simulink model "SimulinkModel"  (R2025b)
settings: Solver=VariableStepAuto  StartTime=0.0  StopTime=3600  FixedStep=0.1  MaxStep=5  MinStep=1  RelTol=0.5e-5  AbsTol=1e-5
values from neighbouring files (symbols this model uses):
  clock_drift_rate = 0.5    [run_simulink.m]    (also in sat_scenario.m)
undefined symbols (not defined in the file or in its folder): accelCorrectionInterval, baroCorrectionInterval, deg, gpsCorrectionInterval, IAU, IMUPropInterval, magCorrectionInterval, R_vec, rad, s, WMM2025
libraries: aerolibtransform2 x6, aerolibconvert2 x2, aerolibutil x2, aerolibsatdyn x1, aerolibnav x1, aerolibgravity2 x1, vrlib x1
settings Model: Creator=abhay  LastModifiedBy=abhay
settings DataIOCC: DatasetSignalFormat=timetable

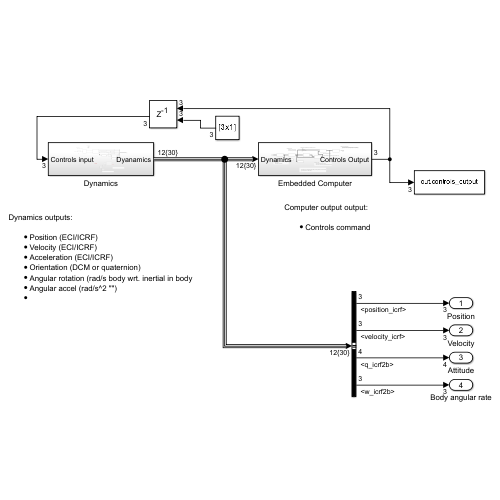
[thumbnail: Simulink's stored preview of the top-level diagram]
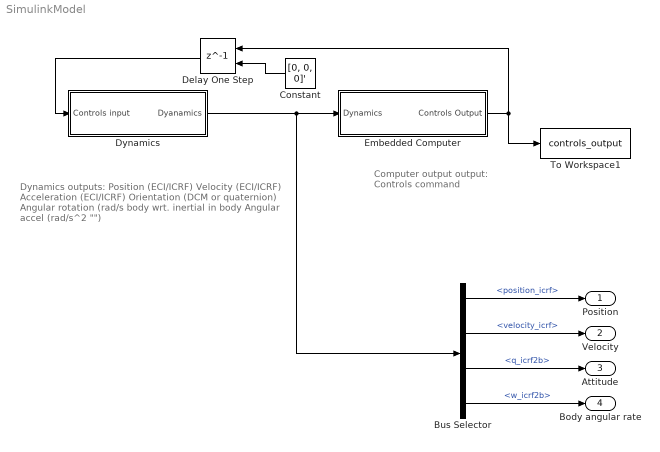
== system SimulinkModel ==
  note: Dynamics outputs:
      |
      | Position (ECI/ICRF)
      | Velocity (ECI/ICRF)
      | Acceleration (ECI/ICRF)
      | Orientation (DCM or quaternion)
      | Angular rotation (rad/s body wrt. inertial in body
      | Angular accel (rad/s^2 "")
  note: Computer output output:
      |
      | Controls command
  Bus Selector : BusSelector  OutputSignals=position_icrf,velocity_icrf,q_icrf2b,w_icrf2b
  Constant : Constant  Value=[0, 0, 0]'
  Delay One Step : Delay  DelayLength=1  InitialConditionSource=Input port
      settings: InputPortMap=u0,p4
  Dynamics : Subsystem
  Embedded Computer : Subsystem
  To Workspace1 : ToWorkspace  VariableName=controls_output  SaveFormat=Timeseries  SampleTime=-1
  Position : Outport
  Velocity : Outport  Port=2
  Attitude : Outport  Port=3
  Body angular rate : Outport  Port=4
  wires:
  Dynamics/1(Dyanamics) -> Bus Selector/1, Embedded Computer/1(Dynamics)
  Embedded Computer/1(Controls Output) -> Delay One Step/1, To Workspace1/1
  Delay One Step/1 -> Dynamics/1(Controls input)
  Constant/1 -> Delay One Step/2
  Bus Selector/1 -> Position/1  "<position_icrf>"
  Bus Selector/2 -> Velocity/1  "<velocity_icrf>"
  Bus Selector/3 -> Attitude/1  "<q_icrf2b>"
  Bus Selector/4 -> Body angular rate/1  "<w_icrf2b>"

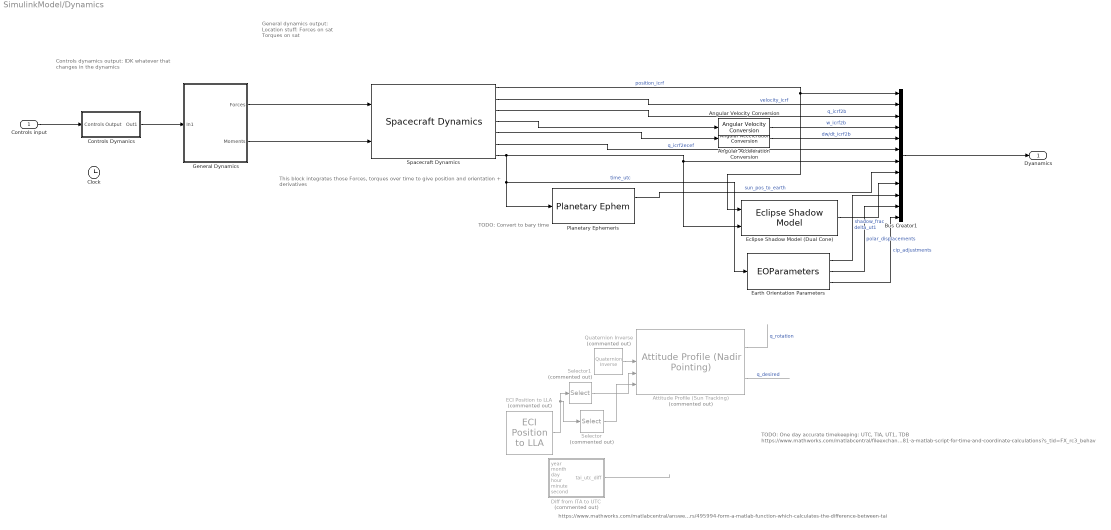
== system SimulinkModel/Dynamics ==
  note: TODO: One day accurate timekeeping: UTC, TIA, UT1, TDB
      |
      | https://www.mathworks.com/matlabcentral/fileexchange/41681-a-matlab-script-for-time-and-coordinate-calculations?s_tid=FX_rc3_behav
  note: TODO: Convert to bary time
  note: https://www.mathworks.com/matlabcentral/answers/495994-form-a-matlab-function-which-calculates-the-difference-between-tai
  note: This block integrates those Forces, torques over time to give position and orientation
      | + derivatives
  note: Controls dynamics output:
      |
      | IDK whatever that changes in the dynamics
  note: General dynamics output:
      |
      | Location stuff:
      | Forces on sat
      | Torques on sat
  Controls input : Inport
  Angular Acceleration Conversion : aerolibconvert2/Angular Acceleration Conversion  IU=deg/s^2  OU=rad/s^2
  Angular Velocity Conversion : aerolibconvert2/Angular Velocity Conversion  IU=deg/s  OU=rad/s
  Attitude Profile (Sun Tracking) : aerolibsatdyn/Attitude Profile (Nadir Pointing)  Commented=on  outputError=on  outputFinalAttitude=on  portFrame=ICRF  pointingMode=Point at celestial body  celestialTarget=Sun  tunablePointing=on  primaryAlignmentSrc=Dialog  primaryAlignment=[0 0 1]  secondaryAlignmentSrc=Dialog  secondaryAlignment=[1 0 0]  constraintFrame=ICRF  primaryConstraintSrc=Dialog  primaryConstraint=[1 0 0]  secondaryConstraintSrc=Dialog  secondaryConstraint=[0 1 0]
      settings: LibrarySourceBlock=|
      | aerolibsatdyn/Attitude Profile
      | (Sun Tracking)
  Bus Creator1 : BusCreator  Inputs=12
  Clock : Clock
  Controls Dymanics : Subsystem
  "Diff from ITA to UTC  " : MATLAB Function  Commented=on  TreatAsAtomicUnit=on
  ECI Position to LLA : aerolibtransform2/ECI Position to LLA  Commented=on  red=IAU-2000/2006  year=2013  month=January  day=1  hour=0  min=0  sec=0  deltaT=Day  errorflag=Error  extraparamflag=on  eunits=Metric (MKS)  earthmodel=WGS84  flat=1/298.257223563  eqradius=6378137
      settings: AttributesFormatString=%<red>
  Earth Orientation Parameters : EOParameters
  Eclipse Shadow Model (Dual Cone) : EclipseShadowModel  timeSource=Port (Julian date)  useEphemerisDateRange=off  zeroCrossing=on
  General Dynamics : Subsystem
  Planetary Ephemeris : PlanetaryEphem  units=m,m/s  target=Sun
  Quaternion Inverse : aerolibutil/Quaternion Inverse  Commented=on
  Selector : Selector  Commented=on  InputPortWidth=3  IndexOptions=Index vector (dialog)  Indices=[3]  OutputSizes=1
  Selector1 : Selector  Commented=on  InputPortWidth=3  IndexOptions=Index vector (dialog)  Indices=[1 2]  OutputSizes=1
  Spacecraft Dynamics : SpacecraftDynamics  startDate=2459581  mass=0.250  inertia=inertia_tensor  semiMajorAxis=6865000  eccentricity=0.0002105  inclination=97.4  raan=0  argPeriapsis=0  trueAnomaly=0  attitude=[0.263360579192421 0.571813128030932 0.494678363680335 0.599136268678053]  attitudeRate=[10 5 2.5]  outputAngAccel=on  outputTransform=on  useDrag=on  useEphemerisDateRange=off  useSRP=on
  Dyanamics : Outport
  wires:
  Controls Dymanics/1(Out1) -> General Dynamics/1(In1)
  General Dynamics/1(Forces) -> Spacecraft Dynamics/1
  General Dynamics/2(Moments) -> Spacecraft Dynamics/2
  Spacecraft Dynamics/1 -> Eclipse Shadow Model (Dual Cone)/1, Bus Creator1/1  "position_icrf"
  Spacecraft Dynamics/2 -> Bus Creator1/2  "velocity_icrf"
  Spacecraft Dynamics/3 -> Bus Creator1/3  "q_icrf2b"
  Spacecraft Dynamics/4 -> Angular Velocity Conversion/1
  Spacecraft Dynamics/5 -> Angular Acceleration Conversion/1
  Spacecraft Dynamics/6 -> Bus Creator1/6  "q_icrf2ecef"
  Spacecraft Dynamics/7 -> Eclipse Shadow Model (Dual Cone)/2, Bus Creator1/7, Planetary Ephemeris/1, Earth Orientation Parameters/1  "time_utc"
  Bus Creator1/1 -> Dyanamics/1
  Controls input/1 -> Controls Dymanics/1(Controls Output)
  ? -> ?
  Angular Velocity Conversion/1 -> Bus Creator1/4  "w_icrf2b"
  Angular Acceleration Conversion/1 -> Bus Creator1/5  "dw/dt_icrf2b"
  Quaternion Inverse/1 -> Attitude Profile (Sun Tracking)/3
  Planetary Ephemeris/1 -> Bus Creator1/8  "sun_pos_to_earth"
  Selector/1 -> Attitude Profile (Sun Tracking)/5
  ECI Position to LLA/1 -> Selector1/1, Selector/1
  Selector1/1 -> Attitude Profile (Sun Tracking)/4
  Attitude Profile (Sun Tracking)/1 -> ?  "q_rotation"
  Attitude Profile (Sun Tracking)/2 -> ?  "q_desired"
  "Diff from ITA to UTC  "/1(tai_utc_diff) -> ?
  Eclipse Shadow Model (Dual Cone)/1 -> Bus Creator1/9  "shadow_frac"
  Earth Orientation Parameters/1 -> Bus Creator1/10  "delta_ut1"
  Earth Orientation Parameters/2 -> Bus Creator1/11  "polar_displacements"
  Earth Orientation Parameters/3 -> Bus Creator1/12  "cip_adjustments"

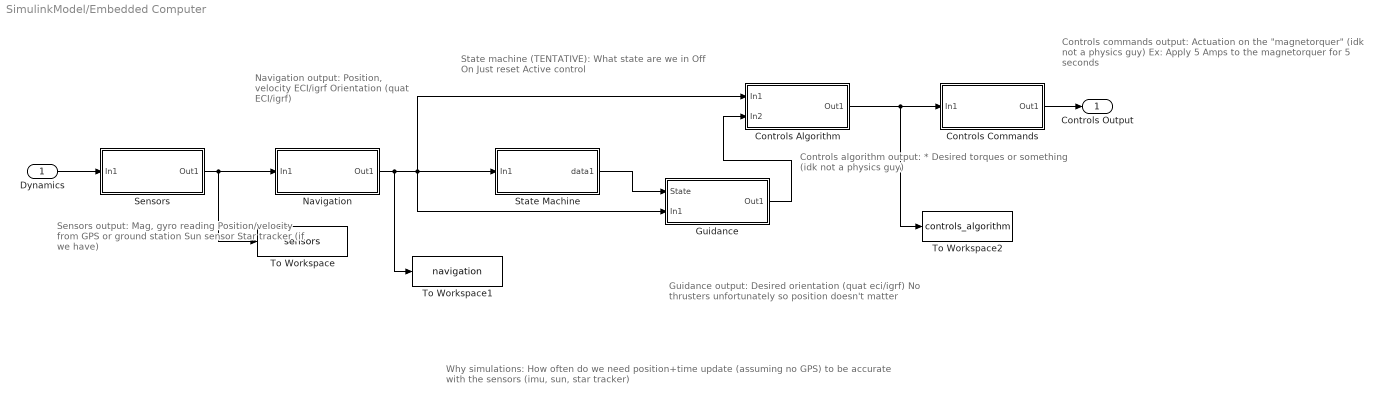
== system SimulinkModel/Embedded Computer ==
  note: Why simulations:
      |
      | How often do we need position+time update (assuming no GPS) to be accurate with the sensors (imu, sun, star tracker)
  note: State machine (TENTATIVE): What state are we in
      | Off
      | On
      | Just reset
      | Active control
  note: Controls commands output:
      | Actuation on the "magnetorquer" (idk not a physics guy)
      | Ex: Apply 5 Amps to the magnetorquer for 5 seconds
  note: Controls algorithm output:
      |
      | * Desired torques or something (idk not a physics guy)
  note: Guidance output:
      | Desired orientation (quat eci/igrf)
      | No thrusters unfortunately so position doesn't matter
  note: Navigation output:
      | Position, velocity ECI/igrf
      | Orientation (quat ECI/igrf)
  note: Sensors output:
      |
      | Mag, gyro reading
      | Position/velocity from GPS or ground station
      | Sun sensor
      | Star tracker (if we have)
  Dynamics : Inport
  Controls Algorithm : Subsystem
  Controls Commands : Subsystem
  Guidance : Subsystem
  Navigation : Subsystem
  Sensors : Subsystem
  State Machine : Subsystem
  To Workspace : ToWorkspace  VariableName=sensors  SaveFormat=Timeseries  SampleTime=-1
  To Workspace1 : ToWorkspace  VariableName=navigation  SaveFormat=Timeseries  SampleTime=-1
  To Workspace2 : ToWorkspace  VariableName=controls_algorithm  SaveFormat=Timeseries  SampleTime=-1
  Controls Output : Outport
  wires:
  Dynamics/1 -> Sensors/1(In1)
  Sensors/1(Out1) -> To Workspace/1, Navigation/1(In1)
  Navigation/1(Out1) -> State Machine/1(In1), Guidance/2(In1), Controls Algorithm/1(In1), To Workspace1/1
  Guidance/1(Out1) -> Controls Algorithm/2(In2)
  Controls Algorithm/1(Out1) -> Controls Commands/1(In1), To Workspace2/1
  Controls Commands/1(Out1) -> Controls Output/1
  State Machine/1(data1) -> Guidance/1(State)

== system SimulinkModel/Dynamics/Controls Dymanics ==
  Controls Output : Inport
  Out1 : Outport
  wires:
  Controls Output/1 -> Out1/1

== system SimulinkModel/Dynamics/General Dynamics ==
  In1 : Inport
  Constant : Constant  Value=[0, 0, 0]'
  Constant1 : Constant  Value=[0, 0, 0]'
  Terminator : Terminator
  Forces : Outport
  Moments : Outport  Port=2
  wires:
  In1/1 -> Terminator/1
  Constant1/1 -> Moments/1
  Constant/1 -> Forces/1

== system SimulinkModel/Embedded Computer/Controls Algorithm ==
  note: *Algorithm: PID, Lya, LQR, etc.
  In1 : Inport
  In2 : Inport  Port=2
  Out1 : Outport
  wires:
  In1/1 -> Out1/1

== system SimulinkModel/Embedded Computer/Controls Commands ==
  note: IDK take desired torques and map to magnetorquer outpit
  In1 : Inport
  Constant : Constant  Value=[0; 0; 0]
  Terminator : Terminator
  Out1 : Outport
  wires:
  In1/1 -> Terminator/1
  Constant/1 -> Out1/1

== system SimulinkModel/Embedded Computer/Guidance ==
  State : Inport
  In1 : Inport  Port=2
  Out1 : Outport
  wires:
  In1/1 -> Out1/1

== system SimulinkModel/Embedded Computer/Navigation ==
  note: Example Q-MEKF I wrote. Use for reference.
      | Isn't robust:
      | * No total orientation through TRIAD, etc.
      | * In NED/ECEF, not ECI
      | *Not robust for a long cycle
  note: Q-MEKF loop:
      | Take in sensors and output state
  In1 : Inport
  Direction Cosine Matrix ECI to ECEF : aerolibtransform2/Direction Cosine Matrix ECI to ECEF  Commented=on  red=IAU-2000/2006  year=2013  month=January  day=1  hour=0  min=0  sec=0  deltaT=None  errorflag=Error  extraparamflag=on
      settings: AttributesFormatString=%<red>
  Earth Orientation Parameters : EOParameters  Commented=on
  Example Q-Mekf : Subsystem  Commented=on
  Nav Init : Subsystem  Commented=on
  Q-MEKF Loop : Subsystem  Commented=on
  Out1 : Outport
  wires:
  In1/1 -> Out1/1
  Nav Init/1(Out1) -> Q-MEKF Loop/2(Q-MEKF k-1)
  Q-MEKF Loop/1(Out1) -> Nav Init/1(In1)
  Earth Orientation Parameters/2 -> Direction Cosine Matrix ECI to ECEF/3
  Earth Orientation Parameters/3 -> Direction Cosine Matrix ECI to ECEF/4

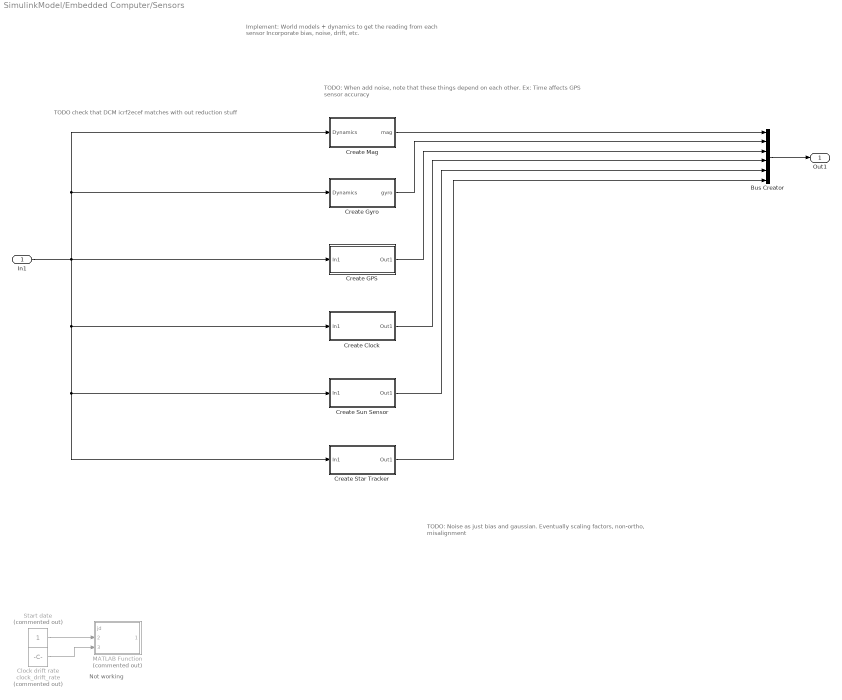
== system SimulinkModel/Embedded Computer/Sensors ==
  note: TODO: When add noise, note that these things depend on each other. Ex: Time affects GPS sensor accuracy
  note: TODO check that DCM icrf2ecef matches with out reduction stuff
  note: TODO:
      | Noise as just bias and gaussian. Eventually scaling factors, non-ortho, misalignment
  note: Not working
  note: Implement:
      | World models + dynamics to get the reading from each sensor
      | Incorporate bias, noise, drift, etc.
  In1 : Inport
  Bus Creator : BusCreator  Inputs=6
  Clock drift rate : Constant  Commented=on  Value=clock_drift_rate
  Create Clock : Subsystem
  Create GPS : Subsystem
  Create Gyro : Subsystem
  Create Mag : Subsystem
  Create Star Tracker : Subsystem
  Create Sun Sensor : Subsystem
  MATLAB Function : MATLAB Function  Commented=on  TreatAsAtomicUnit=on
  Start date : Constant  Commented=on
  Out1 : Outport
  wires:
  Bus Creator/1 -> Out1/1
  Clock drift rate/1 -> MATLAB Function/3(clock_drift_rate)
  Start date/1 -> MATLAB Function/2(startDate)
  In1/1 -> Create Star Tracker/1(In1), Create Sun Sensor/1(In1), Create Clock/1(In1), Create Gyro/1(Dynamics), Create Mag/1(Dynamics), Create GPS/1(In1)
  Create Mag/1(mag) -> Bus Creator/1
  Create Gyro/1(gyro) -> Bus Creator/2
  Create GPS/1(Out1) -> Bus Creator/3
  Create Clock/1(Out1) -> Bus Creator/4
  Create Sun Sensor/1(Out1) -> Bus Creator/5
  Create Star Tracker/1(Out1) -> Bus Creator/6

== system SimulinkModel/Embedded Computer/State Machine ==
  note: State machine: What state are we in
      | Off
      | On
      | Just reset
      | Active control
  In1 : Inport
  Chart : Stateflow chart  Commented=on  TreatAsAtomicUnit=on
  data1 : Outport
  wires:
  In1/1 -> data1/1

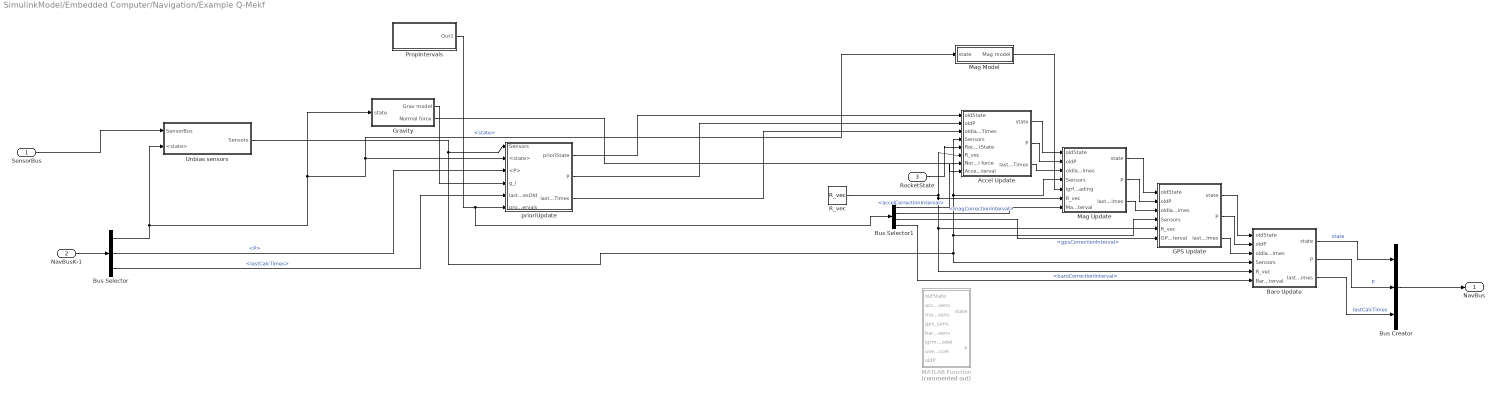
== system SimulinkModel/Embedded Computer/Navigation/Example Q-Mekf ==
  SensorBus : Inport
  NavBusK-1 : Inport  Port=2
  RocketState : Inport  Port=3
  Accel Update : Subsystem
  Baro Update : Subsystem
  Bus Creator : BusCreator  Inputs=3
  Bus Selector : BusSelector  OutputSignals=state,P,lastCalcTimes
  Bus Selector1 : BusSelector  OutputSignals=accelCorrectionInterval,magCorrectionInterval,gpsCorrectionInterval,baroCorrectionInterval
  GPS Update : Subsystem
  Gravity : Subsystem
  MATLAB Function : MATLAB Function  Commented=on  TreatAsAtomicUnit=on
  Mag Model : Subsystem
  Mag Update : Subsystem
  PropIntervals : Subsystem
  R_vec : Constant  Value=R_vec
  Unbias sensors : Subsystem
  prioriUpdate : Subsystem
  NavBus : Outport
  wires:
  R_vec/1 -> Accel Update/6(R_vec), Baro Update/5(R_vec), GPS Update/5(R_vec), Mag Update/6(R_vec)
  GPS Update/3(lastCalcTimes) -> Baro Update/3(oldlastCalcTimes)
  Bus Selector1/1 -> Accel Update/8(Accel Correction Interval)  "<accelCorrectionInterval>"
  Bus Selector/3 -> prioriUpdate/5(lastCalcTimesOld)  "<lastCalcTimes>"
  RocketState/1 -> Accel Update/5(RocketState)
  Bus Creator/1 -> NavBus/1
  Unbias sensors/1(Sensors) -> Baro Update/4(Sensors), Mag Update/4(Sensors), Accel Update/4(Sensors), GPS Update/4(Sensors), prioriUpdate/1(Sensors)
  prioriUpdate/3(lastCalcTimes) -> Accel Update/3(oldlastCalcTimes)
  Bus Selector1/3 -> GPS Update/6(GPS Correction Interval)  "<gpsCorrectionInterval>"
  Bus Selector/2 -> prioriUpdate/3(<P>)  "<P>"
  Bus Selector1/4 -> Baro Update/6(Baro Correction Interval)  "<baroCorrectionInterval>"
  Mag Update/3(lastCalcTimes) -> GPS Update/3(oldlastCalcTimes)
  Bus Selector1/2 -> Mag Update/7(Mag Correction Interval)  "<magCorrectionInterval>"
  Gravity/2(Normal force) -> Accel Update/7(Normal force)
  Accel Update/2(P) -> Mag Update/2(oldP)
  NavBusK-1/1 -> Bus Selector/1
  Accel Update/3(lastCalcTimes) -> Mag Update/3(oldlastCalcTimes)
  Baro Update/1(state) -> Bus Creator/1  "state"
  prioriUpdate/2(P) -> Accel Update/2(oldP)
  PropIntervals/1(Out1) -> Bus Selector1/1, prioriUpdate/6(propIntervals)
  Bus Selector/1 -> Gravity/1(state), prioriUpdate/2(<state>), Mag Model/1(state), Unbias sensors/2(<state>)  "<state>"
  Baro Update/2(P) -> Bus Creator/2  "P"
  Mag Update/2(P) -> GPS Update/2(oldP)
  SensorBus/1 -> Unbias sensors/1(SensorBus)
  Gravity/1(Grav model) -> prioriUpdate/4(g_i)
  GPS Update/2(P) -> Baro Update/2(oldP)
  Mag Update/1(state) -> GPS Update/1(oldState)
  prioriUpdate/1(prioriState) -> Accel Update/1(oldState)
  Baro Update/3(lastCalcTimes) -> Bus Creator/3  "lastCalcTimes"
  GPS Update/1(state) -> Baro Update/1(oldState)
  Accel Update/1(state) -> Mag Update/1(oldState)
  Mag Model/1(Mag model) -> Mag Update/5(igrf_reading)

== system SimulinkModel/Embedded Computer/Navigation/Nav Init ==
  In1 : Inport
  Out1 : Outport
  wires:
  In1/1 -> Out1/1

== system SimulinkModel/Embedded Computer/Navigation/Q-MEKF Loop ==
  Sensors : Inport
  Q-MEKF k-1 : Inport  Port=2
  Bus Selector : BusSelector  Commented=on  OutputSignals=gyro
  Bus Selector1 : BusSelector  Commented=on  OutputSignals=signal1,signal2
  MATLAB Function : MATLAB Function  Commented=on  TreatAsAtomicUnit=on
  Out1 : Outport
  wires:
  Sensors/1 -> Out1/1
  Bus Selector/1 -> ?  "<gyro>"
  Q-MEKF k-1/1 -> Bus Selector1/1
  Bus Selector1/1 -> MATLAB Function/1(gyro)  "<signal1>"
  MATLAB Function/1(q_new) -> ?

== system SimulinkModel/Embedded Computer/Sensors/Create Clock ==
  In1 : Inport
  Bus Selector : BusSelector  OutputSignals=time_utc
  Out1 : Outport
  wires:
  In1/1 -> Bus Selector/1
  Bus Selector/1 -> Out1/1  "<time_utc>"

== system SimulinkModel/Embedded Computer/Sensors/Create GPS ==
  In1 : Inport
  Bus Selector : BusSelector  OutputSignals=q_icrf2ecef,position_icrf
  Matrix Multiply : Product  Multiplication=Matrix(*)
  Quaternions to Direction Cosine Matrix : Quat2Dcm
  Out1 : Outport
  wires:
  In1/1 -> Bus Selector/1
  Bus Selector/1 -> Quaternions to Direction Cosine Matrix/1  "<q_icrf2ecef>"
  Quaternions to Direction Cosine Matrix/1 -> Matrix Multiply/1
  Bus Selector/2 -> Matrix Multiply/2  "<position_icrf>"
  Matrix Multiply/1 -> Out1/1

== system SimulinkModel/Embedded Computer/Sensors/Create Gyro ==
  note: No G's experienced even if grav there
  Dynamics : Inport
  Bus Selector : BusSelector  OutputSignals=w_icrf2b
  Constant1 : Constant  Value=[0, 0, 0]'
  Three-axis Gyroscope : aerolibnav/Three-axis Gyroscope  dtype_g=off  w_g=190  z_g=0.707  g_sf_cc=[1 0 0; 0 1 0; 0 0 1]  g_bias=[0 0 0]  g_sen=[0 0 0]  g_Ts=0  g_rand=off  g_seeds=[23093 23094 23095]  g_pow=[0.0001 0.0001 0.0001]  g_sat="[-inf  -inf  -inf  inf inf inf]"
  gyro : Outport
  wires:
  Three-axis Gyroscope/1 -> gyro/1  "gyro"
  Constant1/1 -> Three-axis Gyroscope/2
  Bus Selector/1 -> Three-axis Gyroscope/1  "<w_icrf2b>"
  Dynamics/1 -> Bus Selector/1

== system SimulinkModel/Embedded Computer/Sensors/Create Mag ==
  Dynamics : Inport
  Bus Selector : BusSelector  OutputSignals=q_icrf2b,position_icrf,q_icrf2ecef
  Demux : Demux  Outputs=2
  Direction Cosine Matrix ECEF to NED : aerolibtransform2/Direction Cosine Matrix ECEF to NED  Commented=on
  ECEF Position to LLA : ECEF2LLA
  Get DCM_NED->Body @ Loc : Subsystem
  Matrix Multiply : Product  Multiplication=Matrix(*)
  Quaternion Rotation : aerolibutil/Quaternion Rotation
  World Magnetic Model : aerolibgravity2/World Magnetic Model  model=WMM2025 (2025-2030)  customFile='WMM2025.COF'  units=Metric (MKS)  time_in=off  month=January  day=1  year=2025  action=Error  h_out=on  dec_out=on  inc_out=on  ti_out=on
  corrupt_mag : MATLAB Function  TreatAsAtomicUnit=on
  mag : Outport
  wires:
  Get DCM_NED->Body @ Loc/1(DCM_NED->Body) -> Matrix Multiply/1
  World Magnetic Model/1 -> Matrix Multiply/2
  Matrix Multiply/1 -> corrupt_mag/1(oldMag)  "mag"
  Quaternion Rotation/1 -> Get DCM_NED->Body @ Loc/3(ECEF Pos), ECEF Position to LLA/1
  ECEF Position to LLA/1 -> Demux/1
  Demux/1 -> World Magnetic Model/2
  Demux/2 -> World Magnetic Model/3
  ECEF Position to LLA/2 -> World Magnetic Model/1
  Dynamics/1 -> Bus Selector/1
  Bus Selector/2 -> Quaternion Rotation/2  "<position_icrf>"
  Bus Selector/3 -> Get DCM_NED->Body @ Loc/2(icrf2ecef), Quaternion Rotation/1  "<q_icrf2ecef>"
  Bus Selector/1 -> Get DCM_NED->Body @ Loc/1(icrf2body)  "<q_icrf2b>"
  corrupt_mag/1(mag) -> mag/1

== system SimulinkModel/Embedded Computer/Sensors/Create Star Tracker ==
  In1 : Inport
  Bus Selector : BusSelector  OutputSignals=q_icrf2b
  Out1 : Outport
  wires:
  In1/1 -> Bus Selector/1
  Bus Selector/1 -> Out1/1  "<q_icrf2b>"

== system SimulinkModel/Embedded Computer/Sensors/Create Sun Sensor ==
  In1 : Inport
  Bus Selector : BusSelector  OutputSignals=q_icrf2b,position_icrf,sun_pos_to_earth,shadow_frac
  Constant : Constant  Value=[0, 0, 0]'
  Matrix Multiply : Product  Multiplication=Matrix(*)
  Normalize Vector : vrlib/Utilities/Normalize Vector  maxzero=0
  Quaternions to Direction Cosine Matrix : Quat2Dcm
  Subtract : Sum  Inputs=+-
  Switch : Switch  Criteria=u2 > Threshold  Threshold=0.5  SaturateOnIntegerOverflow=off  InputSameDT=off
  Out1 : Outport
  wires:
  In1/1 -> Bus Selector/1
  Bus Selector/2 -> Subtract/2  "<position_icrf>"
  Bus Selector/3 -> Subtract/1  "<sun_pos_to_earth>"
  Subtract/1 -> Matrix Multiply/2
  Bus Selector/1 -> Quaternions to Direction Cosine Matrix/1  "<q_icrf2b>"
  Matrix Multiply/1 -> Switch/1
  Bus Selector/4 -> Switch/2  "<shadow_frac>"
  Constant/1 -> Switch/3
  Switch/1 -> Normalize Vector/1
  Quaternions to Direction Cosine Matrix/1 -> Matrix Multiply/1
  Normalize Vector/1 -> Out1/1

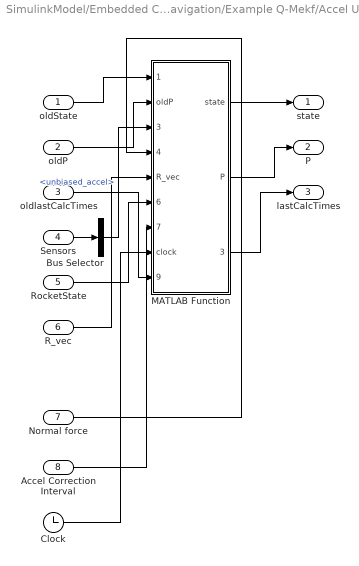
== system SimulinkModel/Embedded Computer/Navigation/Example Q-Mekf/Accel Update ==
  oldState : Inport
  oldP : Inport  Port=2
  oldlastCalcTimes : Inport  Port=3
  Sensors : Inport  Port=4
  RocketState : Inport  Port=5
  R_vec : Inport  Port=6
  Normal force : Inport  Port=7
  Accel Correction Interval : Inport  Port=8
  Bus Selector : BusSelector  OutputSignals=unbiased_accel
  Clock : Clock
  MATLAB Function : MATLAB Function  TreatAsAtomicUnit=on
  state : Outport
  P : Outport  Port=2
  lastCalcTimes : Outport  Port=3
  wires:
  oldState/1 -> MATLAB Function/1(oldState)
  oldP/1 -> MATLAB Function/2(oldP)
  oldlastCalcTimes/1 -> MATLAB Function/9(lastCalcTimesOld)
  Sensors/1 -> Bus Selector/1
  Bus Selector/1 -> MATLAB Function/3(accel_sens)  "<unbiased_accel>"
  R_vec/1 -> MATLAB Function/5(R_vec)
  RocketState/1 -> MATLAB Function/6(RocketState)
  MATLAB Function/1(state) -> state/1
  MATLAB Function/2(P) -> P/1
  Normal force/1 -> MATLAB Function/4(normal_force)
  Accel Correction Interval/1 -> MATLAB Function/7(accelCorrectionInterval)
  Clock/1 -> MATLAB Function/8(clock)
  MATLAB Function/3(lastCalcTimes) -> lastCalcTimes/1

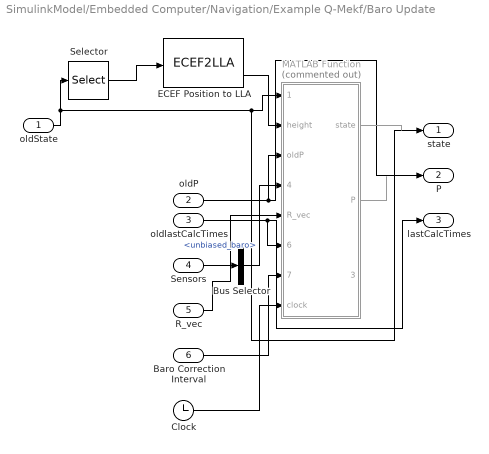
== system SimulinkModel/Embedded Computer/Navigation/Example Q-Mekf/Baro Update ==
  oldState : Inport
  oldP : Inport  Port=2
  oldlastCalcTimes : Inport  Port=3
  Sensors : Inport  Port=4
  R_vec : Inport  Port=5
  Baro Correction Interval : Inport  Port=6
  Bus Selector : BusSelector  OutputSignals=unbiased_baro
  Clock : Clock
  ECEF Position to LLA : ECEF2LLA
  MATLAB Function : MATLAB Function  Commented=on  TreatAsAtomicUnit=on
  Selector : Selector  InputPortWidth=20  IndexOptions=Index vector (dialog)  Indices=[8 9 10]  OutputSizes=1
  state : Outport
  P : Outport  Port=2
  lastCalcTimes : Outport  Port=3
  wires:
  oldState/1 -> Selector/1, state/1, MATLAB Function/1(oldState)
  oldlastCalcTimes/1 -> lastCalcTimes/1, MATLAB Function/6(oldlastCalcTimes)
  oldP/1 -> P/1, MATLAB Function/3(oldP)
  Sensors/1 -> Bus Selector/1
  Bus Selector/1 -> MATLAB Function/4(baro_sens)  "<unbiased_baro>"
  R_vec/1 -> MATLAB Function/5(R_vec)
  MATLAB Function/1(state) -> ?
  MATLAB Function/2(P) -> ?
  Selector/1 -> ECEF Position to LLA/1
  ECEF Position to LLA/2 -> MATLAB Function/2(height)
  Baro Correction Interval/1 -> MATLAB Function/7(baro_correction_interval)
  Clock/1 -> MATLAB Function/8(clock)

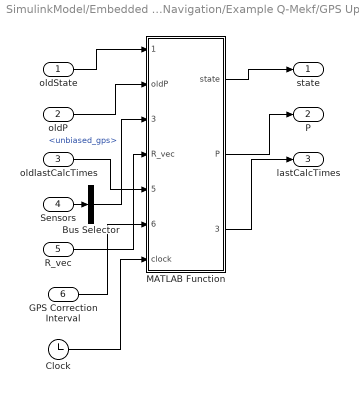
== system SimulinkModel/Embedded Computer/Navigation/Example Q-Mekf/GPS Update ==
  oldState : Inport
  oldP : Inport  Port=2
  oldlastCalcTimes : Inport  Port=3
  Sensors : Inport  Port=4
  R_vec : Inport  Port=5
  GPS Correction Interval : Inport  Port=6
  Bus Selector : BusSelector  OutputSignals=unbiased_gps
  Clock : Clock
  MATLAB Function : MATLAB Function  TreatAsAtomicUnit=on
  state : Outport
  P : Outport  Port=2
  lastCalcTimes : Outport  Port=3
  wires:
  oldState/1 -> MATLAB Function/1(oldState)
  oldP/1 -> MATLAB Function/2(oldP)
  oldlastCalcTimes/1 -> MATLAB Function/5(oldlastCalcTimes)
  MATLAB Function/1(state) -> state/1
  MATLAB Function/2(P) -> P/1
  Sensors/1 -> Bus Selector/1
  Bus Selector/1 -> MATLAB Function/3(gps_sens)  "<unbiased_gps>"
  R_vec/1 -> MATLAB Function/4(R_vec)
  GPS Correction Interval/1 -> MATLAB Function/6(gps_correction_interval)
  Clock/1 -> MATLAB Function/7(clock)
  MATLAB Function/3(lastCalcTimes) -> lastCalcTimes/1

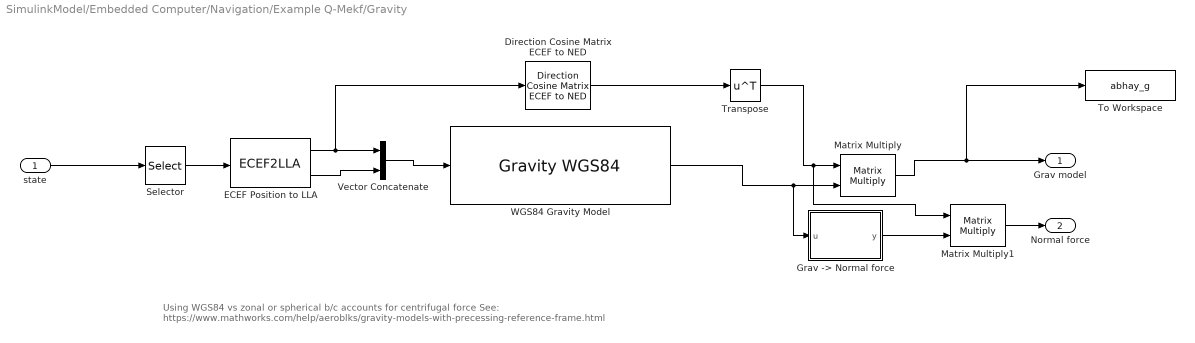
== system SimulinkModel/Embedded Computer/Navigation/Example Q-Mekf/Gravity ==
  note: Using WGS84 vs zonal or spherical b/c accounts for centrifugal force See: https://www.mathworks.com/help/aeroblks/gravity-models-with-precessing-reference-frame.html
  state : Inport
  Direction Cosine Matrix ECEF to NED : aerolibtransform2/Direction Cosine Matrix ECEF to NED
  ECEF Position to LLA : ECEF2LLA
  "Grav -> Normal force" : MATLAB Function  TreatAsAtomicUnit=on
  Matrix Multiply : Product  Multiplication=Matrix(*)
  Matrix Multiply1 : Product  Multiplication=Matrix(*)
  Selector : Selector  InputPortWidth=20  IndexOptions=Index vector (dialog)  Indices=[8 9 10]  OutputSizes=1
  To Workspace : ToWorkspace  VariableName=abhay_g  SaveFormat=Timeseries  SampleTime=-1
  Transpose : Math  Operator=transpose
  Vector Concatenate : Concatenate
  "WGS84 Gravity Model  " : GravityWGS84
  Grav model : Outport
  Normal force : Outport  Port=2
  wires:
  state/1 -> Selector/1
  Selector/1 -> ECEF Position to LLA/1
  "WGS84 Gravity Model  "/1 -> "Grav -> Normal force"/1(u), Matrix Multiply/2
  ECEF Position to LLA/1 -> Direction Cosine Matrix ECEF to NED/1, Vector Concatenate/1
  ECEF Position to LLA/2 -> Vector Concatenate/2
  Vector Concatenate/1 -> "WGS84 Gravity Model  "/1
  Direction Cosine Matrix ECEF to NED/1 -> Transpose/1
  Transpose/1 -> Matrix Multiply1/1, Matrix Multiply/1
  Matrix Multiply/1 -> Grav model/1, To Workspace/1
  "Grav -> Normal force"/1(y) -> Matrix Multiply1/2
  Matrix Multiply1/1 -> Normal force/1

== system SimulinkModel/Embedded Computer/Navigation/Example Q-Mekf/Mag Model ==
  state : Inport
  Demux : Demux  Outputs=3
  Direction Cosine Matrix ECEF to NED : aerolibtransform2/Direction Cosine Matrix ECEF to NED
  ECEF Position to LLA : ECEF2LLA
  International Geomagnetic Reference Field : IGRF  time_in=off  month=January  day=1
      settings: AttributesFormatString=%<generation>
  Matrix Multiply : Product  Multiplication=Matrix(*)
  Selector : Selector  InputPortWidth=20  IndexOptions=Index vector (dialog)  Indices=[8 9 10]  OutputSizes=1
  To uT : Gain  Gain=1.0 / 1000
  Transpose : Math  Operator=transpose
  Vector Concatenate : Concatenate
  Mag model : Outport
  wires:
  International Geomagnetic Reference Field/1 -> To uT/1
  Demux/1 -> International Geomagnetic Reference Field/2
  Demux/2 -> International Geomagnetic Reference Field/3
  Demux/3 -> International Geomagnetic Reference Field/1
  Vector Concatenate/1 -> Demux/1
  To uT/1 -> Matrix Multiply/2
  state/1 -> Selector/1
  Selector/1 -> ECEF Position to LLA/1
  ECEF Position to LLA/1 -> Direction Cosine Matrix ECEF to NED/1, Vector Concatenate/1
  ECEF Position to LLA/2 -> Vector Concatenate/2
  Transpose/1 -> Matrix Multiply/1
  Direction Cosine Matrix ECEF to NED/1 -> Transpose/1
  Matrix Multiply/1 -> Mag model/1

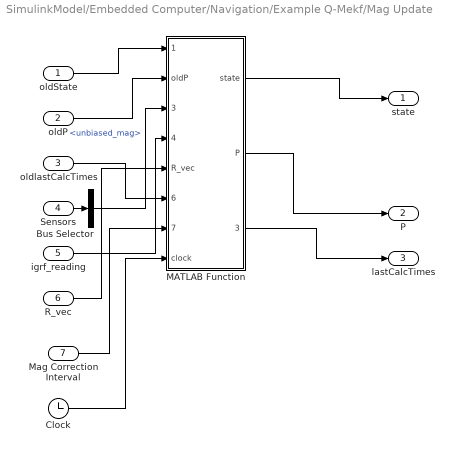
== system SimulinkModel/Embedded Computer/Navigation/Example Q-Mekf/Mag Update ==
  oldState : Inport
  oldP : Inport  Port=2
  oldlastCalcTimes : Inport  Port=3
  Sensors : Inport  Port=4
  igrf_reading : Inport  Port=5
  R_vec : Inport  Port=6
  Mag Correction Interval : Inport  Port=7
  Bus Selector : BusSelector  OutputSignals=unbiased_mag
  Clock : Clock
  MATLAB Function : MATLAB Function  TreatAsAtomicUnit=on
  state : Outport
  P : Outport  Port=2
  lastCalcTimes : Outport  Port=3
  wires:
  oldState/1 -> MATLAB Function/1(oldState)
  oldP/1 -> MATLAB Function/2(oldP)
  oldlastCalcTimes/1 -> MATLAB Function/6(oldlastCalcTimes)
  Sensors/1 -> Bus Selector/1
  Bus Selector/1 -> MATLAB Function/3(mag_sens)  "<unbiased_mag>"
  igrf_reading/1 -> MATLAB Function/4(igrm_model)
  R_vec/1 -> MATLAB Function/5(R_vec)
  MATLAB Function/1(state) -> state/1
  MATLAB Function/2(P) -> P/1
  Mag Correction Interval/1 -> MATLAB Function/7(magCorrectionInterval)
  Clock/1 -> MATLAB Function/8(clock)
  MATLAB Function/3(lastCalcTimes) -> lastCalcTimes/1

== system SimulinkModel/Embedded Computer/Navigation/Example Q-Mekf/PropIntervals ==
  Bus Creator : BusCreator  Inputs=5
  Constant : Constant  Value=IMUPropInterval
  Constant1 : Constant  Value=accelCorrectionInterval
  Constant2 : Constant  Value=magCorrectionInterval
  Constant3 : Constant  Value=gpsCorrectionInterval
  Constant4 : Constant  Value=baroCorrectionInterval
  Out1 : Outport
  wires:
  Constant/1 -> Bus Creator/1  "IMUPropInterval"
  Constant1/1 -> Bus Creator/2  "accelCorrectionInterval"
  Constant2/1 -> Bus Creator/3  "magCorrectionInterval"
  Constant3/1 -> Bus Creator/4  "gpsCorrectionInterval"
  Constant4/1 -> Bus Creator/5  "baroCorrectionInterval"
  Bus Creator/1 -> Out1/1

== system SimulinkModel/Embedded Computer/Navigation/Example Q-Mekf/Unbias sensors ==
  SensorBus : Inport
  <state> : Inport  Port=2
  "Baro Alt -> EcefZ" : Subsystem  Commented=on
  Bus Creator1 : BusCreator  Inputs=5
  Bus Selector1 : BusSelector  OutputSignals=ICM20948.w_ib_B_true,ICM20948.w_ib_B_corr,ICM20948.sf_B_true,ICM20948.sf_B_corr,MMC5983.B_true,MMC5983.B_corr,MAX10S.P_E,MAX10S.P_E_corr,LPS22.P_true,LPS22.P_corr
  Remove Sensor Bias : MATLAB Function  TreatAsAtomicUnit=on
  Sensors : Outport
  wires:
  Remove Sensor Bias/2(unbiased_accel) -> Bus Creator1/2
  Bus Selector1/4 -> Remove Sensor Bias/2(accel_sens)  "<sf_B_corr>"
  Bus Creator1/1 -> Sensors/1
  Remove Sensor Bias/1(unbiased_gyro) -> Bus Creator1/1
  <state>/1 -> Remove Sensor Bias/6(state)
  Remove Sensor Bias/3(unbiased_mag) -> Bus Creator1/3
  Remove Sensor Bias/5(unbiased_baro) -> Bus Creator1/5
  SensorBus/1 -> Bus Selector1/1
  Bus Selector1/2 -> Remove Sensor Bias/1(gyro_sens)  "<w_ib_B_corr>"
  Bus Selector1/9 -> Remove Sensor Bias/5(baro_sens)  "<P_true>"
  Bus Selector1/6 -> Remove Sensor Bias/3(mag_sens)  "<B_corr>"
  Bus Selector1/8 -> Remove Sensor Bias/4(gps_sens)  "<P_E_corr>"
  Remove Sensor Bias/4(unbiased_gps) -> Bus Creator1/4

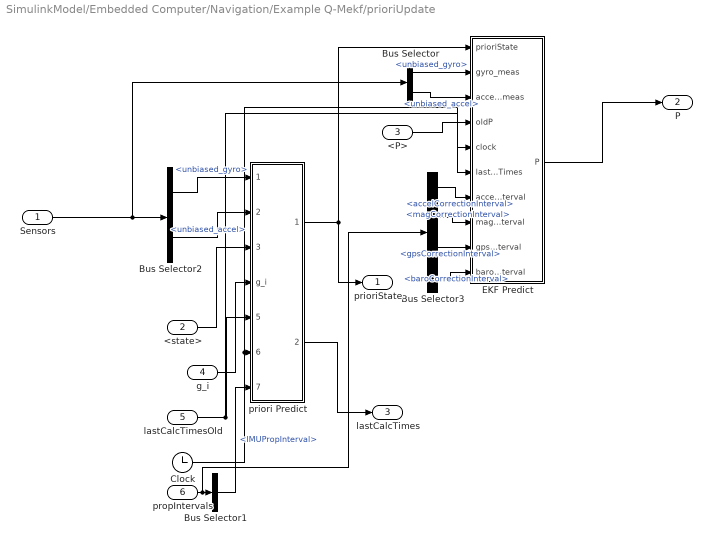
== system SimulinkModel/Embedded Computer/Navigation/Example Q-Mekf/prioriUpdate ==
  Sensors : Inport
  <state> : Inport  Port=2
  <P> : Inport  Port=3
  g_i : Inport  Port=4
  lastCalcTimesOld : Inport  Port=5
  propIntervals : Inport  Port=6
  Bus Selector : BusSelector  OutputSignals=unbiased_gyro,unbiased_accel
  Bus Selector1 : BusSelector  OutputSignals=IMUPropInterval
  Bus Selector2 : BusSelector  OutputSignals=unbiased_gyro,unbiased_accel
  Bus Selector3 : BusSelector  OutputSignals=accelCorrectionInterval,magCorrectionInterval,gpsCorrectionInterval,baroCorrectionInterval
  Clock : Clock
  EKF Predict : MATLAB Function  TreatAsAtomicUnit=on
  priori Predict : MATLAB Function  TreatAsAtomicUnit=on
  prioriState : Outport
  P : Outport  Port=2
  lastCalcTimes : Outport  Port=3
  wires:
  Bus Selector2/2 -> priori Predict/2(accel_meas)  "<unbiased_accel>"
  priori Predict/1(newState) -> EKF Predict/1(prioriState), prioriState/1
  <state>/1 -> priori Predict/3(prevState)
  EKF Predict/1(P) -> P/1
  Sensors/1 -> Bus Selector/1, Bus Selector2/1
  <P>/1 -> EKF Predict/4(oldP)
  g_i/1 -> priori Predict/4(g_i)
  Bus Selector2/1 -> priori Predict/1(gyro_meas)  "<unbiased_gyro>"
  Bus Selector/1 -> EKF Predict/2(gyro_meas)  "<unbiased_gyro>"
  Bus Selector/2 -> EKF Predict/3(accel_meas)  "<unbiased_accel>"
  lastCalcTimesOld/1 -> EKF Predict/6(lastCalcTimes), priori Predict/5(lastCalcTimesOld)
  Clock/1 -> EKF Predict/5(clock), priori Predict/6(clock)
  propIntervals/1 -> Bus Selector3/1, Bus Selector1/1
  Bus Selector1/1 -> priori Predict/7(imuPropInterval)  "<IMUPropInterval>"
  priori Predict/2(lastCalcTimes) -> lastCalcTimes/1
  Bus Selector3/1 -> EKF Predict/7(accelCorrectionInterval)  "<accelCorrectionInterval>"
  Bus Selector3/2 -> EKF Predict/8(magCorrectionInterval)  "<magCorrectionInterval>"
  Bus Selector3/3 -> EKF Predict/9(gpsCorrectionInterval)  "<gpsCorrectionInterval>"
  Bus Selector3/4 -> EKF Predict/10(baroCorrectionInterval)  "<baroCorrectionInterval>"

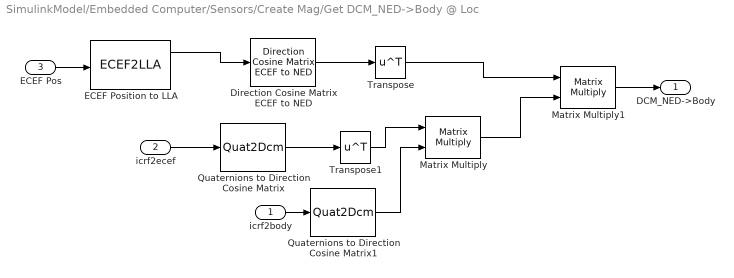
== system SimulinkModel/Embedded Computer/Sensors/Create Mag/Get DCM_NED->Body @ Loc ==
  icrf2body : Inport
  icrf2ecef : Inport  Port=2
  ECEF Pos : Inport  Port=3
  Direction Cosine Matrix ECEF to NED : aerolibtransform2/Direction Cosine Matrix ECEF to NED
  ECEF Position to LLA : ECEF2LLA
  Matrix Multiply : Product  Multiplication=Matrix(*)
  Matrix Multiply1 : Product  Multiplication=Matrix(*)
  Quaternions to Direction Cosine Matrix : Quat2Dcm
  Quaternions to Direction Cosine Matrix1 : Quat2Dcm
  Transpose : Math  Operator=transpose
  Transpose1 : Math  Operator=transpose
  DCM_NED->Body : Outport
  wires:
  ECEF Pos/1 -> ECEF Position to LLA/1
  ECEF Position to LLA/1 -> Direction Cosine Matrix ECEF to NED/1
  Direction Cosine Matrix ECEF to NED/1 -> Transpose/1
  Transpose/1 -> Matrix Multiply1/1
  icrf2ecef/1 -> Quaternions to Direction Cosine Matrix/1
  Quaternions to Direction Cosine Matrix/1 -> Transpose1/1
  icrf2body/1 -> Quaternions to Direction Cosine Matrix1/1
  Transpose1/1 -> Matrix Multiply/1
  Quaternions to Direction Cosine Matrix1/1 -> Matrix Multiply/2
  Matrix Multiply/1 -> Matrix Multiply1/2
  Matrix Multiply1/1 -> DCM_NED->Body/1

== system SimulinkModel/Embedded Computer/Navigation/Example Q-Mekf/Unbias sensors/Baro Alt -> EcefZ ==
  Baro : Inport
  state : Inport  Port=2
  ECEF Position to LLA : ECEF2LLA
  LLA to ECEF Position : LLA2ECEF
  Selector : Selector  InputPortWidth=20  IndexOptions=Index vector (dialog)  Indices=[8 9 10]  OutputSizes=1
  Selector1 : Selector  InputPortWidth=3  IndexOptions=Index vector (dialog)  Indices=[3]  OutputSizes=1
  Baro ECEF_Z : Outport
  wires:
  state/1 -> Selector/1
  Selector/1 -> ECEF Position to LLA/1
  ECEF Position to LLA/1 -> LLA to ECEF Position/1
  Baro/1 -> LLA to ECEF Position/2
  LLA to ECEF Position/1 -> Selector1/1
  Selector1/1 -> Baro ECEF_Z/1

== matlab function SimulinkModel/Embedded Computer/Navigation/Example Q-Mekf/MATLAB Function ==
  data: oldState input; accel_sens input; mag_sens input; gps_sens input; baro_sens input; igrm_model input; state output; P output; use_accel input; oldP input
function [state, P] = fcn(oldState, accel_sens, mag_sens, gps_sens, baro_sens, igrm_model, use_accel, oldP)


%if use_accel
    %[residual, H, R] = measAccelMag(oldState, accel_sens, mag_sens, gps_sens, baro_sens, igrm_model);
%else
    %[residual, H, R] = measMag(oldState, mag_sens, gps_sens, baro_sens, igrm_model);

%end

%disp("Use accel")
%use_accel
%disp("Residual")
%if size(residual, 1) == 2
%residual

%[state, P] = EKFCalculationsAndErrorInject(residual, H, oldP, R, oldState);

state = oldState;
P = oldP;

== matlab function SimulinkModel/Embedded Computer/Navigation/Example Q-Mekf/Mag Update/MATLAB Function ==
  data: oldState input; oldP input; state output; mag_sens input; igrm_model input; R_vec input; P output; oldlastCalcTimes input; magCorrectionInterval input; clock input; lastCalcTimes output
function [state, P, lastCalcTimes] = fcn(oldState, oldP, mag_sens, igrm_model, R_vec, oldlastCalcTimes, magCorrectionInterval, clock)
lastCalcTimes = oldlastCalcTimes;
if clock - oldlastCalcTimes(3) >= magCorrectionInterval

    q = oldState(1:4)';
    
    H_mag = [skewSymmetric(quat2dcm(q) * igrm_model), zeros(3), zeros(3), zeros(3), zeros(3), eye(3), zeros(3, 1)];
    
    h_mag = quat2dcm(q) * igrm_model;
    
    R = diag(R_vec(4:6));
    
    [state, P] = residualErrorInject(oldState, oldP, mag_sens, H_mag, h_mag, R);
else
    state = oldState;
    P = oldP;
end

== matlab function SimulinkModel/Embedded Computer/Navigation/Example Q-Mekf/GPS Update/MATLAB Function ==
  data: oldState input; oldP input; state output; gps_sens input; R_vec input; P output; oldlastCalcTimes input; gps_correction_interval input; clock input; lastCalcTimes output
function [state, P, lastCalcTimes] = fcn(oldState, oldP, gps_sens, R_vec, oldlastCalcTimes, gps_correction_interval, clock)

lastCalcTimes = oldlastCalcTimes;

if clock - lastCalcTimes(4) >= gps_correction_interval

    H_gps = [zeros(3), zeros(3), eye(3), zeros(3), zeros(3), zeros(3), zeros(3, 1)];
    
    h_gps = oldState(8:10);
    
    R = diag(R_vec(7:9));
    
    [state, P] = residualErrorInject(oldState, oldP, gps_sens, H_gps, h_gps, R);
else
    state = oldState;
    P = oldP;
end

== matlab function SimulinkModel/Embedded Computer/Navigation/Example Q-Mekf/Baro Update/MATLAB Function ==
  data: oldState input; height input; oldP input; state output; baro_sens input; R_vec input; P output; oldlastCalcTimes input; baro_correction_interval input; clock input; lastCalcTimes output
function [state, P, lastCalcTimes] = fcn(oldState, height, oldP, baro_sens, R_vec, oldlastCalcTimes, baro_correction_interval, clock)
% TODO subject of future research
%if clock - lastCalcTimes(4) >= gps_correction_interval
% TODO these are here b/c I don't know how to matlab, otherwise erase
P0 = 101325;
L  = 0.0065;
T0  = 288.15;
M   = 0.0289644;
R   = 8.3144598;
g_e = 9.80665;

H_baro = [zeros(1, 3), zeros(1, 3), [0, 0, 0], zeros(1, 3), zeros(1, 3), zeros(1, 3), 1];

h_baro = P0 * (1 - (L * height) / T0)^(g_e*M / (R*L));

%disp("Recreation of baro")
%disp(h_baro)
%disp("Actual baro")
%disp(baro_sens)

R = R_vec(10);

[state, P] = residualErrorInject(oldState, oldP, baro_sens, H_baro, h_baro, R);

== matlab function SimulinkModel/Embedded Computer/Navigation/Example Q-Mekf/Accel Update/MATLAB Function ==
  data: oldState input; oldP input; state output; accel_sens input; normal_force input; R_vec input; P output; RocketState input; accelCorrectionInterval input; clock input; lastCalcTimesOld input; lastCalcTimes output
function [state, P, lastCalcTimes] = fcn(oldState, oldP, accel_sens, normal_force, R_vec, RocketState, accelCorrectionInterval, clock, lastCalcTimesOld)

% TODO: One day model the accelerometer using drag forces, etc.
q = oldState(1:4)';
lastCalcTimes = lastCalcTimesOld;

if RocketState == 0 && clock - accelCorrectionInterval >= lastCalcTimesOld(2)
    H_accel = [skewSymmetric(quat2dcm(q) * normal_force), zeros(3), zeros(3), zeros(3), eye(3), zeros(3), zeros(3, 1)];
    
    h_accel = quat2dcm(q) * normal_force;
    
    R = diag(R_vec(1:3));
    
    [state, P] = residualErrorInject(oldState, oldP, accel_sens, H_accel, h_accel, R);
else
    state = oldState;
    P = oldP;
end

== matlab function SimulinkModel/Embedded Computer/Navigation/Example Q-Mekf/Gravity/Grav -> Normal force ==
  data: u input; y output
function y = fcn(u)

y = [u(1); u(2); -1.0 * u(3)];

== stateflow chart SimulinkModel/Embedded Computer/State Machine/Chart ==
  data: data input; data1 output

== matlab function SimulinkModel/Embedded Computer/Sensors/MATLAB Function ==
  data: jd input; new_jd output; startDate input; clock_drift_rate input
function new_jd = fcn(jd, startDate, clock_drift_rate)
    curr_dt = datetime(jd,'convertfrom','juliandate');
    elapsed_time = curr_dt - startDate;
    new_dt = DAY(elapsed_time) + days(elapsed_time) * clock_drift_rate;
    new_jd = juliandate(new_dt);

== matlab function SimulinkModel/Embedded Computer/Navigation/Q-MEKF Loop/MATLAB Function ==
  data: gyro input; state_vec_prev input; q_new output
function q_new = fcn(gyro, state_vec_prev)

attitude_q = state_vec_prev(1:4);

rot_vec_norm = norm(gyro);

qdot = [cos(rot_vec_norm),
        gyro(1) * sin(rot_vec_norm),
        gyro(2) * sin(rot_vec_norm),
        gyro(3) * sin(rot_vec_norm)];

q_new = attitude_q * qdot;

== matlab function SimulinkModel/Dynamics/Diff from ITA to UTC   ==
  data: year input; tai_utc_diff output; month input; day input; hour input; minute input; second input
function tai_utc_diff = calculateTAI_UTC(year, month, day, hour, minute, second) 
    % List of leap seconds added to UTC since 1972 
    leap_seconds = { 
        datetime(1972, 7, 1), 10; 
        datetime(1973, 1, 1), 11; 
        datetime(1974, 1, 1), 12; 
        datetime(1975, 1, 1), 13; 
        datetime(1976, 1, 1), 14; 
        datetime(1977, 1, 1), 15; 
        datetime(1978, 1, 1), 16; 
        datetime(1979, 1, 1), 17; 
        datetime(1980, 1, 1), 18; 
        datetime(1981, 7, 1), 19; 
        datetime(1982, 7, 1), 20; 
        datetime(1983, 7, 1), 21; 
        datetime(1985, 7, 1), 22; 
        datetime(1988, 1, 1), 23; 
        datetime(1990, 1, 1), 24; 
        datetime(1991, 1, 1), 25; 
        datetime(1992, 7, 1), 26; 
        datetime(1993, 7, 1), 27; 
        datetime(1994, 7, 1), 28; 
        datetime(1996, 1, 1), 29; 
        datetime(1997, 7, 1), 30; 
        datetime(1999, 1, 1), 31; 
        datetime(2006, 1, 1), 32; 
        datetime(2009, 1, 1), 33; 
        datetime(2012, 7, 1), 34; 
        datetime(2015, 7, 1), 35; 
        datetime(2017, 1, 1), 36; 
        datetime(2023, 1, 1), 37; 
    }; 
    % Create a datetime object for the input date 
    input_date = datetime(year, month, day, hour, minute, second); 
    % Initialize TAI-UTC difference 
    tai_utc_diff = 10; 
    % Loop through leap seconds and find the applicable difference 
    for i = 1:size(leap_seconds, 1) 
        if input_date >= leap_seconds{i, 1} 
            tai_utc_diff = leap_seconds{i, 2}; 
        else
            break; 
        end 
    end
end 

% Example: Calculate TAI-UTC difference for January 1, 2024, at 12:00:00 
diff = calculateTAI_UTC(2024, 1, 1, 12, 0, 0); 
fprintf('TAI-UTC difference: %d seconds\n', diff);

== matlab function SimulinkModel/Embedded Computer/Sensors/Create Mag/corrupt_mag ==
  data: oldMag input; mag output
function mag = fcn(oldMag)

mag = oldMag;

== matlab function SimulinkModel/Embedded Computer/Navigation/Example Q-Mekf/Unbias sensors/Remove Sensor Bias ==
  data: gyro_sens input; accel_sens input; unbiased_gyro output; unbiased_accel output; mag_sens input; gps_sens input; baro_sens input; state input; unbiased_mag output; unbiased_gps output; unbiased_baro output
function [unbiased_gyro, unbiased_accel, unbiased_mag, unbiased_gps, unbiased_baro] = fcn(gyro_sens, accel_sens, mag_sens, gps_sens, baro_sens, state)

unbiased_gyro = gyro_sens - state(11:13);
unbiased_accel = accel_sens - state(14:16);
unbiased_mag = mag_sens - state(17:19);
unbiased_gps = gps_sens;
unbiased_baro = baro_sens - state(20);



%unbiased_gyro = gyro_sens;
%unbiased_mag = mag_sens;
%unbiased_accel = accel_sens;
%unbiased_baro = baro_sens;

== matlab function SimulinkModel/Embedded Computer/Navigation/Example Q-Mekf/prioriUpdate/priori Predict ==
  data: gyro_meas input; newState output; accel_meas input; prevState input; g_i input; lastCalcTimesOld input; clock input; imuPropInterval input; lastCalcTimes output
function [newState, lastCalcTimes] = fcn(gyro_meas, accel_meas, prevState, g_i, lastCalcTimesOld, clock, imuPropInterval)
lastCalcTimes = lastCalcTimesOld;

if clock - lastCalcTimesOld(1) > imuPropInterval
    dt = clock - max(lastCalcTimesOld);
    newState = prioriPropagation(gyro_meas, accel_meas, dt, prevState, g_i);
    lastCalcTimes(1) = clock;
else
    newState = prevState;
end

== matlab function SimulinkModel/Embedded Computer/Navigation/Example Q-Mekf/prioriUpdate/EKF Predict ==
  data: prioriState input; P output; gyro_meas input; accel_meas input; oldP input; clock input; lastCalcTimes input; accelCorrectionInterval input; magCorrectionInterval input; gpsCorrectionInterval input; baroCorrectionInterval input
function P = fcn(prioriState, gyro_meas, accel_meas, oldP, clock, lastCalcTimes, accelCorrectionInterval, magCorrectionInterval, gpsCorrectionInterval, baroCorrectionInterval)

if clock - lastCalcTimes(2) > accelCorrectionInterval || clock - lastCalcTimes(3) > magCorrectionInterval || clock - lastCalcTimes(4) > gpsCorrectionInterval || clock - lastCalcTimes(5) > baroCorrectionInterval
    dt = clock - max(lastCalcTimes(2:5));

    stateTransitionMatrix = createProcessModel(prioriState, gyro_meas, accel_meas, dt);
    
    Q_d = createProcessNoise(dt);
    
    P = stateTransitionMatrix * oldP * transpose(stateTransitionMatrix) + Q_d;
else
    P = oldP;
end
